simulink model "last_test2_rapport"  (Simulink 7.1)
settings: Solver=ode3  StartTime=0.0  StopTime=2000  FixedStep=0.1  RelTol=1e-3
undefined symbols (not defined in the file or in its folder): kalmanfilter4
libraries: fordypningsprosjekt x4
settings Model: Creator=anderga  LastModifiedBy=anders
settings OptimizationCC: SimCompilerOptimization=On

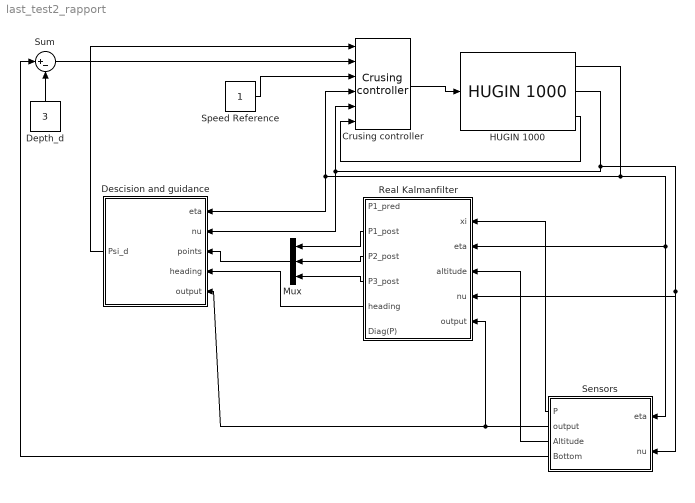
== system last_test2_rapport ==
  Crusing controller : fordypningsprosjekt/Crusing controller  SystemSampleTime=-1  Kp_u=10  Ki_u=3  Kp_c=100  Kd_c=50  Kp_d=50  Kp2_d=20  Kd_d=20
  Depth_d : Constant  Orientation=up  Value=3  OutDataType=sfix(16)  OutScaling=2^0
  Descision and guidance : Subsystem  Orientation=left  AncestorBlock=fordypningsprosjekt/Look-ahead guidance
  HUGIN 1000 : fordypningsprosjekt/HUGIN 1000  SystemSampleTime=-1  eta_0=[-30 -30 0 0 0 0]  nu_0=[0 0 0 0 0 0]  c_on_off=on  beta_c=-45  V_c=0.3
  Mux : Mux  Orientation=left  Inputs=3
  Real Kalmanfilter : Subsystem  Orientation=left  AncestorBlock=fordypningsprosjekt/Real Kalmanfilter
  Sensors : Subsystem  Orientation=left  AncestorBlock=fordypningsprosjekt/Sensors
  Speed Reference : Constant  OutDataType=sfix(16)  OutScaling=2^0
  Sum : Sum  Inputs=|+-  OutDataType=sfix(16)  OutScaling=2^0
  wires:
  Crusing controller/1 -> HUGIN 1000/1
  HUGIN 1000/1 -> Real Kalmanfilter/2(eta), Sensors/1(eta), Crusing controller/4, Descision and guidance/1(eta)
  HUGIN 1000/2 -> Crusing controller/5, Descision and guidance/2(nu), Sensors/2(nu), Real Kalmanfilter/4(nu)
  HUGIN 1000/3 -> Crusing controller/6
  Sensors/1(P) -> Real Kalmanfilter/1(xi)
  Sensors/2(output) -> Real Kalmanfilter/5(output), Descision and guidance/5(output)
  Sensors/3(Altitude) -> Real Kalmanfilter/3(altitude)
  Depth_d/1 -> Sum/2
  Sensors/4(Bottom) -> Sum/1
  Sum/1 -> Crusing controller/2
  Speed Reference/1 -> Crusing controller/3
  Descision and guidance/1(Psi_d) -> Crusing controller/1
  Real Kalmanfilter/5(heading) -> Descision and guidance/4(heading)
  Real Kalmanfilter/2(P1_post) -> Mux/1
  Real Kalmanfilter/3(P2_post) -> Mux/2
  Real Kalmanfilter/4(P3_post) -> Mux/3
  Mux/1 -> Descision and guidance/3(points)

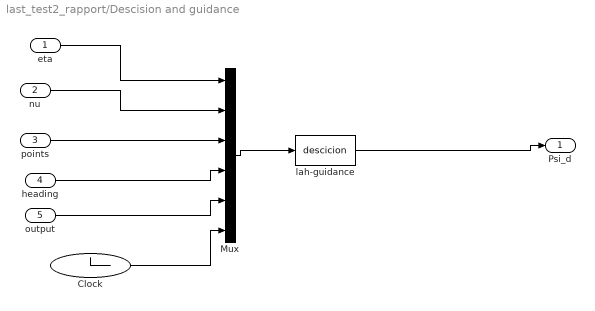
== system last_test2_rapport/Descision and guidance ==
  eta : Inport  OutDataType=sfix(16)  OutScaling=2^0
  nu : Inport  Port=2  OutDataType=sfix(16)  OutScaling=2^0
  points : Inport  Port=3  OutDataType=sfix(16)  OutScaling=2^0
  heading : Inport  Port=4  OutDataType=sfix(16)  OutScaling=2^0
  output : Inport  Port=5  OutDataType=sfix(16)  OutScaling=2^0
  Clock : Clock
  Mux : Mux  Inputs=6
  lah-guidance : MATLABFcn  MATLABFcn=descicion  OutputDimensions=1
  Psi_d : Outport  OutDataType=sfix(16)  OutScaling=2^0
  wires:
  heading/1 -> Mux/4
  points/1 -> Mux/3
  eta/1 -> Mux/1
  nu/1 -> Mux/2
  Mux/1 -> lah-guidance/1
  lah-guidance/1 -> Psi_d/1
  output/1 -> Mux/5
  Clock/1 -> Mux/6

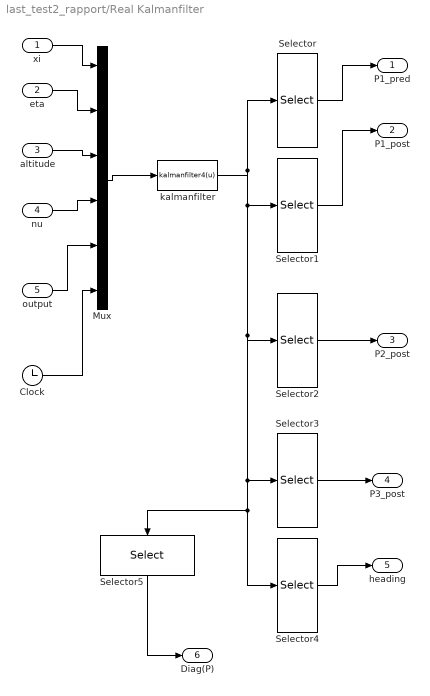
== system last_test2_rapport/Real Kalmanfilter ==
  xi : Inport  OutDataType=sfix(16)  OutScaling=2^0
  eta : Inport  Port=2  OutDataType=sfix(16)  OutScaling=2^0
  altitude : Inport  Port=3  OutDataType=sfix(16)  OutScaling=2^0
  nu : Inport  Port=4  OutDataType=sfix(16)  OutScaling=2^0
  output : Inport  Port=5  OutDataType=sfix(16)  OutScaling=2^0
  Clock : Clock
      settings: Decimation=10
  Mux : Mux  Inputs=6
  Selector : Selector  InputPortWidth=17  IndexOptions=Index vector (dialog)  Indices=[1:3]  OutputSizes=1
  Selector1 : Selector  InputPortWidth=17  IndexOptions=Index vector (dialog)  Indices=4:6  OutputSizes=1
  Selector2 : Selector  InputPortWidth=17  IndexOptions=Index vector (dialog)  Indices=7:9  OutputSizes=1
  Selector3 : Selector  InputPortWidth=17  IndexOptions=Index vector (dialog)  Indices=10:12  OutputSizes=1
  Selector4 : Selector  InputPortWidth=17  IndexOptions=Index vector (dialog)  Indices=13  OutputSizes=1
  Selector5 : Selector  Orientation=down  InputPortWidth=17  IndexOptions=Index vector (dialog)  Indices=14:17  OutputSizes=1
  kalmanfilter : MATLABFcn  MATLABFcn=kalmanfilter4(u)  OutputDimensions=17
  P1_pred : Outport  OutDataType=sfix(16)  OutScaling=2^0
  P1_post : Outport  Port=2  OutDataType=sfix(16)  OutScaling=2^0
  P2_post : Outport  Port=3  OutDataType=sfix(16)  OutScaling=2^0
  P3_post : Outport  Port=4  OutDataType=sfix(16)  OutScaling=2^0
  heading : Outport  Port=5  OutDataType=sfix(16)  OutScaling=2^0
  Diag(P) : Outport  Port=6  OutDataType=sfix(16)  OutScaling=2^0
  wires:
  output/1 -> Mux/5
  Mux/1 -> kalmanfilter/1
  nu/1 -> Mux/4
  altitude/1 -> Mux/3
  eta/1 -> Mux/2
  xi/1 -> Mux/1
  kalmanfilter/1 -> Selector/1, Selector1/1, Selector2/1, Selector3/1, Selector4/1, Selector5/1
  Selector/1 -> P1_pred/1
  Selector1/1 -> P1_post/1
  Selector2/1 -> P2_post/1
  Selector3/1 -> P3_post/1
  Selector4/1 -> heading/1
  Clock/1 -> Mux/6
  Selector5/1 -> Diag(P)/1

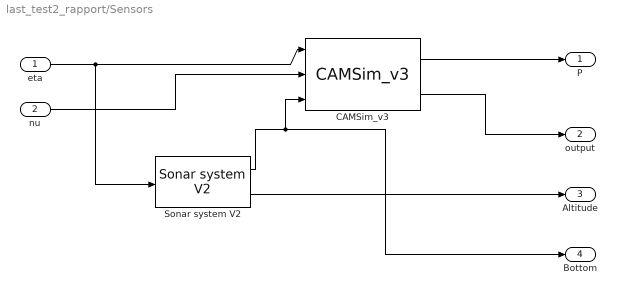
== system last_test2_rapport/Sensors ==
  eta : Inport  OutDataType=sfix(16)  OutScaling=2^0
  nu : Inport  Port=2  OutDataType=sfix(16)  OutScaling=2^0
  CAMSim_v3 : fordypningsprosjekt/CAMSim_v3  SystemSampleTime=-1  noise=on  variance=0.01
      link override MATLAB Fcn: MATLABFcn=camsim3
  Sonar system V2 : fordypningsprosjekt/Sonar system V2  SystemSampleTime=-1  sea_bottom=-40
  P : Outport  OutDataType=sfix(16)  OutScaling=2^0
  output : Outport  Port=2  OutDataType=sfix(16)  OutScaling=2^0
  Altitude : Outport  Port=3  OutDataType=sfix(16)  OutScaling=2^0
  Bottom : Outport  Port=4  OutDataType=sfix(16)  OutScaling=2^0
  wires:
  eta/1 -> Sonar system V2/1, CAMSim_v3/1
  nu/1 -> CAMSim_v3/2
  Sonar system V2/1 -> Bottom/1, CAMSim_v3/3
  Sonar system V2/2 -> Altitude/1
  CAMSim_v3/1 -> P/1
  CAMSim_v3/2 -> output/1
